simulink model "SSI_RT"  (R2020b)
settings: Solver=FixedStepAuto  StartTime=0.0  StopTime=inf  RelTol=1e-3
undefined symbols (not defined in the file): Serial_Port, Standard_Devices
libraries: sldrtlib x2
settings Model: SimulationMode=external  Creator=pavlo  LastModifiedBy=pavlo
settings SolverCC: DecoupledContinuousIntegration=on  MinimalZcImpactIntegration=on
settings DataIOCC: ReturnWorkspaceOutputs=off
settings DebuggingCC: ArithmeticOperatorsInVariantConditions=warning
settings SFSimCC: SimUseLocalCustomCode=off  CustomCodeUndefinedFunction=UseInterfaceOnly
settings RTWCC: Description=Simulink Desktop Real-Time  SystemTargetFile=sldrt.tlc  TemplateMakefile=sldrt.tmf  RTWUseLocalCustomCode=off  RTWCompilerOptimization=on
settings CodeAppCC: MaxIdLength=95
settings SimulinkDesktopRealTimeCC: TargetPreCompLibLocation=D:\MATLAB R2020b\toolbox\sldrt\lib\win64

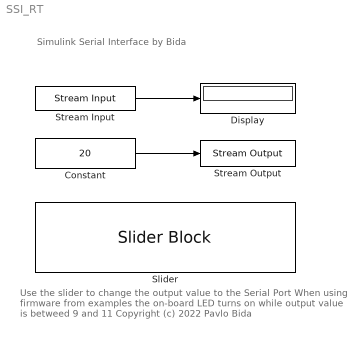
== system SSI_RT ==
  note: Use the slider to change the output value to the Serial Port
      |
      | When using firmware from examples
      | the on-board LED turns on while output value is betweed 9 and 11
      |
      | Copyright (c) 2022 Pavlo Bida
  note: Simulink Serial Interface by Bida
  Constant : Constant  Value=20  OutDataTypeStr=single
  Display : Display
      settings: Format=decimal (Stored Integer)  Decimation=3
  Slider : SliderBlock  ScaleMax=20
  Stream Input : sldrtlib/Stream Input  SampleTime=0.01  MaxMissedTicks=10  ShowMissedTicks=off  YieldWhenWaiting=off  DrvName=Standard_Devices/Serial_Port  DrvAddress=4  DrvOptions=[115200 8 0 0 0 0 0 0]  DataTypes='single'  FormatString='%f'  Terminator={'\r', '\n', '\0'}  ShowReady=off  ShowError=off
      settings: AttributesFormatString=Serial Port [4]  SourceProductBaseCode=WT
  Stream Output : sldrtlib/Stream Output  SampleTime=0.1  MaxMissedTicks=10  ShowMissedTicks=off  YieldWhenWaiting=off  DrvName=Standard_Devices/Serial_Port  DrvAddress=4  DrvOptions=[115200 8 0 0 0 0 0 0]  PortSizes=1  FormatString='%g\r\n'  ShowReady=off  ShowError=off  InitialValue=[]  FinalValue=[]
      settings: AttributesFormatString=Serial Port [4]  SourceProductBaseCode=WT
  wires:
  Stream Input/1 -> Display/1
  Constant/1 -> Stream Output/1
